simulink model "lab4_2"  (R2014b)
settings: Solver=ode45  StartTime=0.0  StopTime=5  RelTol=1e-3
values from neighbouring files (symbols this model uses):
  Lo = cell2mat(num)    [lab4_1.m]
  Lr = Mo    [lab4_1.m]
  Mo = cell2mat(den)    [lab4_1.m]
  Mr = [ 1 0 0 0 ]*L1 - Lo    [lab4_1.m]
libraries: simulink x2
settings Model: Creator=StudentPA  LastModifiedBy=StudentPA

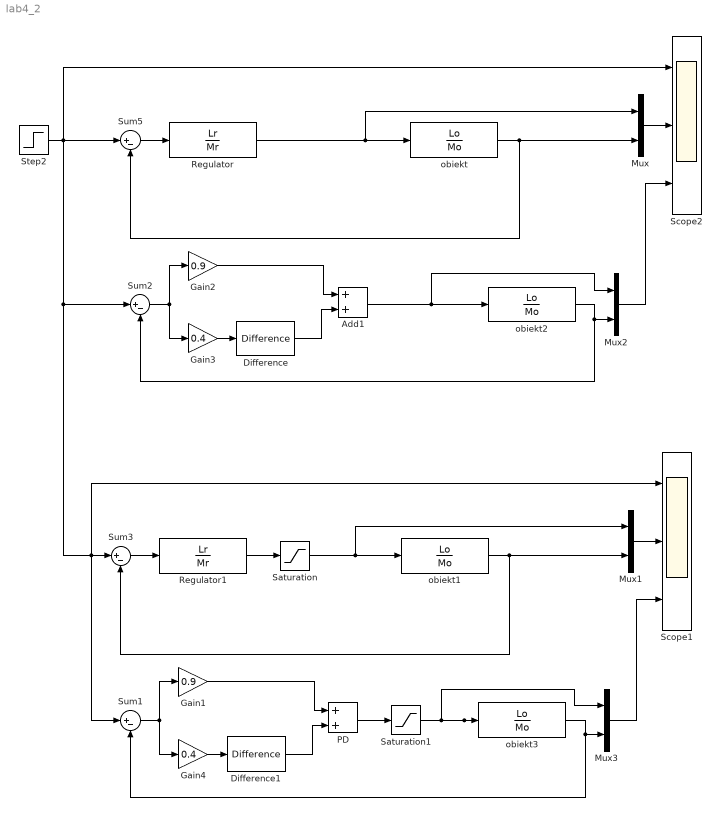
== system lab4_2 ==
  Add1 : Sum
  Difference : simulink/Discrete/Difference  ICPrevInput=0.0  InputProcessing=Inherited  OutMin=[]  OutMax=[]  OutDataType=fixdt(1, 16)  OutScaling=2^-10  DoSatur=off
  Difference1 : simulink/Discrete/Difference  ICPrevInput=0.0  InputProcessing=Inherited  OutMin=[]  OutMax=[]  OutDataType=fixdt(1, 16)  OutScaling=2^-10  DoSatur=off
  Gain1 : Gain  Gain=0.9
  Gain2 : Gain  Gain=0.9
  Gain3 : Gain  Gain=0.4
  Gain4 : Gain  Gain=0.4
  Mux{,1..3} (4 alike) : Mux  Inputs=2
  PD : Sum
  Regulator : DiscreteTransferFcn  Numerator=Lr  Denominator=Mr
  Regulator1 : DiscreteTransferFcn  Numerator=Lr  Denominator=Mr
  Saturation : Saturate  UpperLimit=2  LowerLimit=-2
  Saturation1 : Saturate  UpperLimit=2  LowerLimit=-2
  Scope1 : Scope  NumInputPorts=3
      settings: ShowLegends=on  YMin=0~-5~-5  YMax=2~5~5
  Scope2 : Scope  NumInputPorts=3
      settings: ShowLegends=on  YMin=0~-5~-5  YMax=2~5~5  SaveName=ScopeData2
  Step2 : Step  Time=0.1  SampleTime=0.1
  Sum{1..3,5} (4 alike) : Sum  Inputs=|+-
  obiekt{,1..3} (4 alike) : DiscreteTransferFcn  Numerator=Lo  Denominator=Mo
  wires:
  Regulator/1 -> Mux/1, obiekt/1
  Sum5/1 -> Regulator/1
  obiekt/1 -> Sum5/2, Mux/2
  Mux/1 -> Scope2/2
  Sum2/1 -> Gain3/1, Gain2/1
  Difference/1 -> Add1/2
  Gain2/1 -> Add1/1
  Add1/1 -> Mux2/1, obiekt2/1
  Gain3/1 -> Difference/1
  Regulator1/1 -> Saturation/1
  Sum3/1 -> Regulator1/1
  obiekt1/1 -> Sum3/2, Mux1/2
  Mux1/1 -> Scope1/2
  Sum1/1 -> Gain4/1, Gain1/1
  Step2/1 -> Sum5/1, Sum2/1, Sum3/1, Sum1/1, Scope1/1, Scope2/1
  Difference1/1 -> PD/2
  Gain1/1 -> PD/1
  PD/1 -> Saturation1/1
  Gain4/1 -> Difference1/1
  Saturation/1 -> Mux1/1, obiekt1/1
  obiekt2/1 -> Sum2/2, Mux2/2
  Mux2/1 -> Scope2/3
  Saturation1/1 -> obiekt3/1, Mux3/1
  obiekt3/1 -> Sum1/2, Mux3/2
  Mux3/1 -> Scope1/3
